simulink model "LF_V15_Delay_Perfect"  (Simulink 7.9)
settings: Solver=ode45  StartTime=0.0  StopTime=100*20e-9  RelTol=1e-3
PreLoadFcn:
  | LF_V15_Param;
values from neighbouring files (symbols this model uses):
  Cnt_CPS = 10    [LF_V15_Param.m]
  Exp_ST = 1/Exp_SF    (= 0.002)    [LF_V15_Param.m]
  Kd2 = 0.004    [LF_V15_Param.m]
  Ki2 = 0.03    [LF_V15_Param.m]
  Kp2 = 0.25    [LF_V15_Param.m]
  Reg_En = (2^Err_Acc_Len)-1    (= 511)    [LF_V15_Param.m]
  Saw_CPS = 100    [LF_V15_Param.m]
libraries: xbsIndex_r4 x273
(part 1 of 2)
settings Model: Creator=jbmervin  LastModifiedBy=Sen_Hema

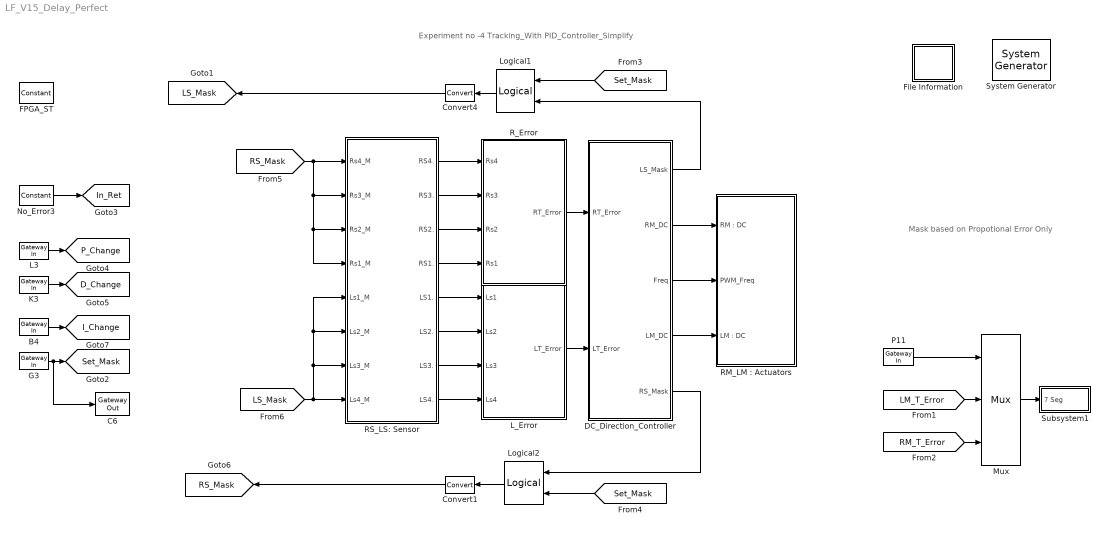
== system LF_V15_Delay_Perfect ==
  note: Experiment no -4 Tracking_With PID_Controller_Simplify
  note: Mask based on Propotional Error Only
  " System Generator" : xbsIndex_r4/ System Generator  Tag=genX  xilinxfamily=spartan3e  part=xc3s100e  speed=-4  package=cp132  synthesis_tool=XST  clock_wrapper=Clock Enables  directory=./LF_V15  proj_type=Project Navigator  Synth_file=XST Defaults  Impl_file=ISE Defaults  testbench=off  simulink_period=20e-9  sysclk_period=20  dcm_input_clock_period=10  incr_netlist=off  trim_vbits=Everywhere in SubSystem  dbl_ovrd=According to Block Masks  core_generation=According to Block Masks  run_coregen=off  deprecated_control=off  eval_field=0  block_type=sysgen
  B4 : xbsIndex_r4/Gateway In  gui_display_data_type=Boolean  arith_type=Boolean  n_bits=1  bin_pt=0  preci_type=Single  exp_width=8  frac_width=24  quantization="Round  (unbiased: +/- Inf)"  overflow=Saturate  period=InPorts_ST  dbl_ovrd=off  timing_constraint=None  locs_specified=on  LOCs={'B4'}  UseAsADC=off  ADCChannel='1'  inherit_from_input=off  hdl_port=on  block_type=gatewayin
  C6 : xbsIndex_r4/Gateway Out  inherit_from_input=off  hdl_port=on  timing_constraint=None  locs_specified=on  LOCs={'C6'}  UseAsDAC=off  DACChannel='1'  block_type=gatewayout
  Convert1 : xbsIndex_r4/Convert  gui_display_data_type=Boolean  arith_type=Boolean  n_bits=16  bin_pt=14  float_type=Single  exp_bits=8  fraction_bits=24  quantization=Truncate  overflow=Wrap  en=off  latency=0  dbl_ovrd=off  pipeline=off  block_type=convert
  Convert4 : xbsIndex_r4/Convert  gui_display_data_type=Boolean  arith_type=Boolean  n_bits=16  bin_pt=14  float_type=Single  exp_bits=8  fraction_bits=24  quantization=Truncate  overflow=Wrap  en=off  latency=0  dbl_ovrd=off  pipeline=off  block_type=convert
  DC_Direction_Controller : Subsystem
  FPGA_ST : xbsIndex_r4/Constant  const=1  gui_display_data_type=Fixed-point  arith_type=Unsigned  n_bits=1  bin_pt=0  preci_type=Single  exp_width=8  frac_width=24  explicit_period=on  period=FPGA_ST  equ=P=C  opselect=C  inp2=PCIN>>17  opr=+  inp1=P  carry=CIN  dbl_ovrd=off  block_type=constant
  File Information : Subsystem
      mask Display:
      | fprintf('','COMMENT: begin icon graphics');
      | patch([24.425 34.54 41.54 48.54 55.54 41.54 31.425 24.425 ],[32.77 32.77 39.77 32.77 39.77 39.77 39.77 32.77 ],[0.965 0.951 0.755 ]);
      | patch([31.425 41.54 34.54 24.425 31.425 ],[25.77 25.77 32.77 32.77 25.77 ],[0.95 0.93 0.15 ]);
      | patch([24.425 34.54 41.54 31.425 24.425 ],[18.77 18.77 25.77 25.77 18.77 ],[0.965 0.951 0.755 ]);
      | patch([31.425 55.54 48.54 41.54 34.54 24.425 31.425 ],[11.77 11.77 18.77 11.77 18.77 18.77 11.77 ],[0.95 0.93 0.15 ]);
      | fprintf('','COMMENT: end icon graphics');
      | fprintf('','COMMENT: end icon text');
  G3 : xbsIndex_r4/Gateway In  gui_display_data_type=Boolean  arith_type=Boolean  n_bits=1  bin_pt=0  preci_type=Single  exp_width=8  frac_width=24  quantization="Round  (unbiased: +/- Inf)"  overflow=Saturate  period=InPorts_ST  dbl_ovrd=off  timing_constraint=None  locs_specified=on  LOCs={'G3'}  UseAsADC=off  ADCChannel='1'  inherit_from_input=off  hdl_port=on  block_type=gatewayin
  K3 : xbsIndex_r4/Gateway In  gui_display_data_type=Boolean  arith_type=Boolean  n_bits=1  bin_pt=0  preci_type=Single  exp_width=8  frac_width=24  quantization="Round  (unbiased: +/- Inf)"  overflow=Saturate  period=InPorts_ST  dbl_ovrd=off  timing_constraint=None  locs_specified=on  LOCs={'K3'}  UseAsADC=off  ADCChannel='1'  inherit_from_input=off  hdl_port=on  block_type=gatewayin
  L3 : xbsIndex_r4/Gateway In  gui_display_data_type=Boolean  arith_type=Boolean  n_bits=1  bin_pt=0  preci_type=Single  exp_width=8  frac_width=24  quantization="Round  (unbiased: +/- Inf)"  overflow=Saturate  period=InPorts_ST  dbl_ovrd=off  timing_constraint=None  locs_specified=on  LOCs={'L3'}  UseAsADC=off  ADCChannel='1'  inherit_from_input=off  hdl_port=on  block_type=gatewayin
  L_Error : Subsystem
  Logical1 : xbsIndex_r4/Logical  logical_function=OR  inputs=2  en=off  latency=0  precision=User Defined  arith_type=Unsigned  n_bits=1  bin_pt=0  align_bp=on  dbl_ovrd=off  block_type=logical
  Logical2 : xbsIndex_r4/Logical  logical_function=OR  inputs=2  en=off  latency=0  precision=User Defined  arith_type=Unsigned  n_bits=1  bin_pt=0  align_bp=on  dbl_ovrd=off  block_type=logical
  Mux : xbsIndex_r4/Mux  inputs=2  en=off  latency=0  precision=Full  arith_type=Unsigned  n_bits=16  bin_pt=14  quantization=Truncate  overflow=Wrap  dbl_ovrd=off  block_type=mux
  No_Error3 : xbsIndex_r4/Constant  const=1  gui_display_data_type=Fixed-point  arith_type=Unsigned  n_bits=1  bin_pt=0  preci_type=Single  exp_width=8  frac_width=24  explicit_period=on  period=Exp_ST  equ=P=C  opselect=C  inp2=PCIN>>17  opr=+  inp1=P  carry=CIN  dbl_ovrd=off  block_type=constant
  P11 : xbsIndex_r4/Gateway In  gui_display_data_type=Boolean  arith_type=Boolean  n_bits=1  bin_pt=0  preci_type=Single  exp_width=8  frac_width=24  quantization="Round  (unbiased: +/- Inf)"  overflow=Saturate  period=20e-9  dbl_ovrd=off  timing_constraint=None  locs_specified=on  LOCs={'P11'}  UseAsADC=off  ADCChannel='1'  inherit_from_input=off  hdl_port=on  block_type=gatewayin
  "RM_LM : Actuators" : Subsystem
  RS_LS: Sensor : Subsystem
  R_Error : Subsystem
  Subsystem1 : Subsystem
  tag scope: D_Change=global, I_Change=global, In_Ret=global, LS_Mask=global, P_Change=global, RS_Mask=global, Set_Mask=global
  wires:
  RS_LS: Sensor/1(RS4.) -> R_Error/1(Rs4)
  RS_LS: Sensor/2(RS3.) -> R_Error/2(Rs3)
  RS_LS: Sensor/3(RS2.) -> R_Error/3(Rs2)
  RS_LS: Sensor/4(RS1.) -> R_Error/4(Rs1)
  RS_LS: Sensor/5(LS1.) -> L_Error/1(Ls1)
  RS_LS: Sensor/6(LS2.) -> L_Error/2(Ls2)
  RS_LS: Sensor/7(LS3.) -> L_Error/3(Ls3)
  RS_LS: Sensor/8(LS4.) -> L_Error/4(Ls4)
  DC_Direction_Controller/3(Freq) -> "RM_LM : Actuators"/2(PWM_Freq)
  DC_Direction_Controller/2(RM_DC) -> "RM_LM : Actuators"/1("RM : DC")
  DC_Direction_Controller/4(LM_DC) -> "RM_LM : Actuators"/3("LM : DC")
  R_Error/1(RT_Error) -> DC_Direction_Controller/1(RT_Error)
  L_Error/1(LT_Error) -> DC_Direction_Controller/2(LT_Error)
  DC_Direction_Controller/5(RS_Mask) -> Logical2/1
  L3/1 -> [P_Change]
  K3/1 -> [D_Change]
  B4/1 -> [I_Change]
  DC_Direction_Controller/1(LS_Mask) -> Logical1/2
  [Set_Mask] -> Logical1/1
  G3/1 -> [Set_Mask], C6/1
  [Set_Mask] -> Logical2/2
  No_Error3/1 -> [In_Ret]
  Logical1/1 -> Convert4/1
  Logical2/1 -> Convert1/1
  [RS_Mask] -> RS_LS: Sensor/1(Rs4_M), RS_LS: Sensor/2(Rs3_M), RS_LS: Sensor/3(Rs2_M), RS_LS: Sensor/4(Rs1_M)
  [LS_Mask] -> RS_LS: Sensor/8(Ls4_M), RS_LS: Sensor/7(Ls3_M), RS_LS: Sensor/5(Ls1_M), RS_LS: Sensor/6(Ls2_M)
  Convert4/1 -> [LS_Mask]
  Convert1/1 -> [RS_Mask]
  Mux/1 -> Subsystem1/1(7 Seg)
  P11/1 -> Mux/1
  [LM_T_Error] -> Mux/2
  [RM_T_Error] -> Mux/3

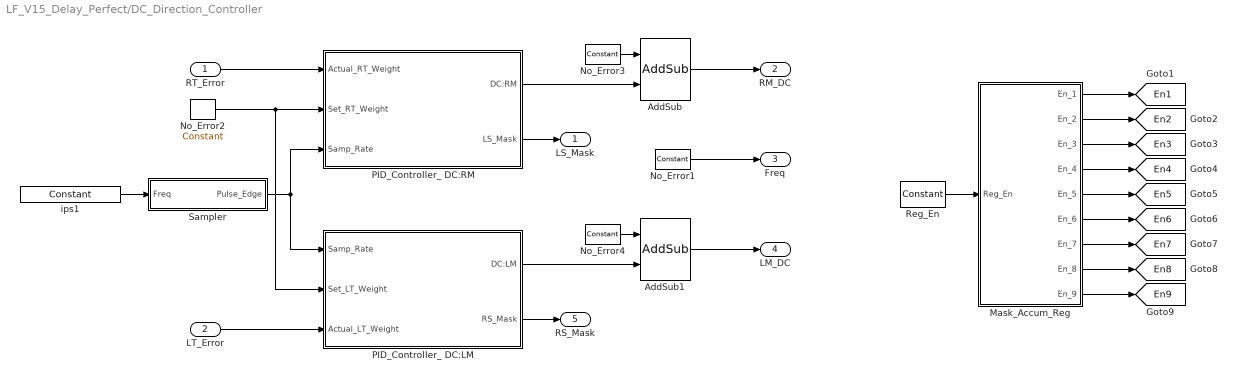
== system LF_V15_Delay_Perfect/DC_Direction_Controller ==
  RT_Error : Inport
  LT_Error : Inport  Port=2
  AddSub : xbsIndex_r4/AddSub  mode=Addition  use_carryin=off  use_carryout=off  en=off  latency=0  precision=Full  arith_type=Unsigned  n_bits=25  bin_pt=20  quantization=Truncate  overflow=Wrap  dbl_ovrd=off  use_behavioral_HDL=off  hw_selection=Fabric  pipelined=off  block_type=addsub
  AddSub1 : xbsIndex_r4/AddSub  mode=Addition  use_carryin=off  use_carryout=off  en=off  latency=0  precision=Full  arith_type=Unsigned  n_bits=25  bin_pt=20  quantization=Truncate  overflow=Wrap  dbl_ovrd=off  use_behavioral_HDL=off  hw_selection=Fabric  pipelined=off  block_type=addsub
  Mask_Accum_Reg : Subsystem
  No_Error1 : xbsIndex_r4/Constant  const=Saw_CPS  gui_display_data_type=Fixed-point  arith_type=Unsigned  n_bits=7  bin_pt=0  preci_type=Single  exp_width=8  frac_width=24  explicit_period=on  period=Exp_ST  equ=P=C  opselect=C  inp2=PCIN>>17  opr=+  inp1=P  carry=CIN  dbl_ovrd=off  block_type=constant
  No_Error2 : xbsIndex_r4/Constant  const=0  gui_display_data_type=Fixed-point  arith_type=Unsigned  n_bits=1  bin_pt=0  preci_type=Single  exp_width=8  frac_width=24  explicit_period=on  period=Exp_ST  equ=P=C  opselect=C  inp2=PCIN>>17  opr=+  inp1=P  carry=CIN  dbl_ovrd=off  block_type=constant
  No_Error3 : xbsIndex_r4/Constant  const=1  gui_display_data_type=Fixed-point  arith_type=Unsigned  n_bits=1  bin_pt=0  preci_type=Single  exp_width=8  frac_width=24  explicit_period=on  period=Exp_ST  equ=P=C  opselect=C  inp2=PCIN>>17  opr=+  inp1=P  carry=CIN  dbl_ovrd=off  block_type=constant
  No_Error4 : xbsIndex_r4/Constant  const=1  gui_display_data_type=Fixed-point  arith_type=Unsigned  n_bits=1  bin_pt=0  preci_type=Single  exp_width=8  frac_width=24  explicit_period=on  period=Exp_ST  equ=P=C  opselect=C  inp2=PCIN>>17  opr=+  inp1=P  carry=CIN  dbl_ovrd=off  block_type=constant
  PID_Controller_ DC:LM : Subsystem
  PID_Controller_ DC:RM : Subsystem
  Reg_En : xbsIndex_r4/Constant  const=Reg_En  gui_display_data_type=Fixed-point  arith_type=Unsigned  n_bits=9  bin_pt=0  preci_type=Single  exp_width=8  frac_width=24  explicit_period=on  period=Exp_ST  equ=P=C  opselect=C  inp2=PCIN>>17  opr=+  inp1=P  carry=CIN  dbl_ovrd=off  block_type=constant
  Sampler : Subsystem
  ips1 : xbsIndex_r4/Constant  const=Cnt_CPS  gui_display_data_type=Fixed-point  arith_type=Unsigned  n_bits=27  bin_pt=0  preci_type=Single  exp_width=8  frac_width=24  explicit_period=on  period=Exp_ST  equ=P=C  opselect=C  inp2=PCIN>>17  opr=+  inp1=P  carry=CIN  dbl_ovrd=off  block_type=constant
  LS_Mask : Outport
  RM_DC : Outport  Port=2
  Freq : Outport  Port=3
  LM_DC : Outport  Port=4
  RS_Mask : Outport  Port=5
  tag scope: En1=global, En2=global, En3=global, En4=global, En5=global, En6=global, En7=global, En8=global, En9=global
  wires:
  No_Error1/1 -> Freq/1
  RT_Error/1 -> PID_Controller_ DC:RM/1(Actual_RT_Weight)
  PID_Controller_ DC:RM/1(DC:RM) -> AddSub/2
  PID_Controller_ DC:LM/1(DC:LM) -> AddSub1/2
  No_Error4/1 -> AddSub1/1
  No_Error3/1 -> AddSub/1
  PID_Controller_ DC:RM/2(LS_Mask) -> LS_Mask/1
  PID_Controller_ DC:LM/2(RS_Mask) -> RS_Mask/1
  Sampler/1(Pulse_Edge) -> PID_Controller_ DC:RM/3(Samp_Rate), PID_Controller_ DC:LM/1(Samp_Rate)
  ips1/1 -> Sampler/1(Freq)
  No_Error2/1 -> PID_Controller_ DC:RM/2(Set_RT_Weight), PID_Controller_ DC:LM/2(Set_LT_Weight)
  AddSub1/1 -> LM_DC/1
  AddSub/1 -> RM_DC/1
  Mask_Accum_Reg/1(En_1) -> [En1]
  Mask_Accum_Reg/2(En_2) -> [En2]
  Mask_Accum_Reg/3(En_3) -> [En3]
  Mask_Accum_Reg/4(En_4) -> [En4]
  Mask_Accum_Reg/5(En_5) -> [En5]
  Mask_Accum_Reg/6(En_6) -> [En6]
  Mask_Accum_Reg/7(En_7) -> [En7]
  Mask_Accum_Reg/8(En_8) -> [En8]
  Mask_Accum_Reg/9(En_9) -> [En9]
  Reg_En/1 -> Mask_Accum_Reg/1("Reg_En ")
  LT_Error/1 -> PID_Controller_ DC:LM/3(Actual_LT_Weight)

== system LF_V15_Delay_Perfect/File Information ==
  note: System Identification - I ( Free Oscillation - Theta Vs Time )
  note: Expirement No -I
  note: Dynamics and Control an Enthralling Journey with Aero Thrust Pendulem
  note: _________________________________________________________________________________________________________________
  note: The Aero Thrust Pendulem is set to oscillate freely and the values of Thetas are sampled at a rate faster than the Period of oscillation
  note: Sampling Time: Sec
  note: The front end of the experiment is designed in Python by Adithya (Team Member) - This front end dynamically captures the theta and displays as a graph on the Computer Screen
      | and Simultaneously it stores the values of theta as a CSV file on the computer.  Note:  Since the initial position is considered as zero Theta. The forward positions are accounted as
      |  (1,2,3,.......60.....70....180)  and Simillarly reverse positions are accounted as (359,358......180)
  note: Method to read the CSV file
  note: Details of Front End Tool
  note: Details of Xilinx File......
  note: This Files Detrmines Theta from the Help of Signals Comming from the Encoder ( A, B, Z (not used)) and sends then theta values (datas) through all the four channels . These Channels communicate
      | the external devices through the RS232 Protocol. Simultaneously the datas are transmitted to four DAC channels Voltage ranging from ( 0V - 3.3V) for display on a CRO. In addition the datas are...
      | Displayed on a  Seven Segment LED Display avaliable on the FPGA Module...........................................................................................................................................................................................
  note: When the pendulum oscillates freely we see that the datas are recorded as ( 60....10...5....0....358.....340.....320...300) and so on .... but this will not give a visual picture of osillations
      | so we need to convert the theta as given. ( if {Theta > 180} then {Theta = (Theta - 360)}, else {Theta=Theta})...............................................................................................................

== system LF_V15_Delay_Perfect/L_Error ==
  Ls1 : Inport
  Ls2 : Inport  Port=2
  Ls3 : Inport  Port=3
  Ls4 : Inport  Port=4
  AddSub1 : xbsIndex_r4/AddSub  mode=Addition  use_carryin=off  use_carryout=off  en=off  latency=0  precision=User Defined  arith_type=Unsigned  n_bits=2  bin_pt=0  quantization=Truncate  overflow=Wrap  dbl_ovrd=off  use_behavioral_HDL=off  hw_selection=Fabric  pipelined=off  block_type=addsub
  AddSub2 : xbsIndex_r4/AddSub  mode=Addition  use_carryin=off  use_carryout=off  en=off  latency=0  precision=User Defined  arith_type=Unsigned  n_bits=4  bin_pt=0  quantization=Truncate  overflow=Wrap  dbl_ovrd=off  use_behavioral_HDL=off  hw_selection=Fabric  pipelined=off  block_type=addsub
  AddSub3 : xbsIndex_r4/AddSub  mode=Addition  use_carryin=off  use_carryout=off  en=off  latency=0  precision=User Defined  arith_type=Unsigned  n_bits=4  bin_pt=0  quantization=Truncate  overflow=Wrap  dbl_ovrd=off  use_behavioral_HDL=off  hw_selection=Fabric  pipelined=off  block_type=addsub
  LT_Error : Outport
  wires:
  AddSub2/1 -> LT_Error/1
  AddSub1/1 -> AddSub2/2
  AddSub3/1 -> AddSub2/1
  Ls1/1 -> AddSub1/2
  Ls2/1 -> AddSub1/1
  Ls3/1 -> AddSub3/2
  Ls4/1 -> AddSub3/1

== system LF_V15_Delay_Perfect/RM_LM : Actuators ==
  "RM : DC" : Inport
  PWM_Freq : Inport  Port=2
  "LM : DC" : Inport  Port=3
  L_Actuator : Subsystem
  RM_LM: F_R_PWM_Generator : Subsystem
  R_Actuators : Subsystem
  wires:
  "RM : DC"/1 -> RM_LM: F_R_PWM_Generator/1(RM:DC)
  "LM : DC"/1 -> RM_LM: F_R_PWM_Generator/2(LM:DC)
  PWM_Freq/1 -> RM_LM: F_R_PWM_Generator/3(RM_LM:PWM_Freq)
  RM_LM: F_R_PWM_Generator/1(RM: F_PWM) -> R_Actuators/1("RM : F_PWM")
  RM_LM: F_R_PWM_Generator/4(LM: F_PWM) -> L_Actuator/2(LM: F_PWM)
  RM_LM: F_R_PWM_Generator/3(LM: R_PWM) -> L_Actuator/1(LM: R_PWM)
  RM_LM: F_R_PWM_Generator/2(RM: R_PWM) -> R_Actuators/2(RM :R_ PWM)

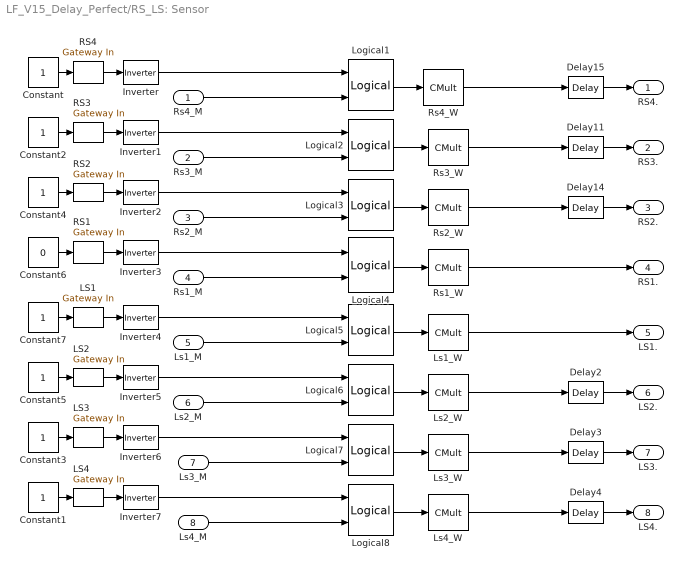
== system LF_V15_Delay_Perfect/RS_LS: Sensor ==
  Rs4_M : Inport
  Rs3_M : Inport  Port=2
  Rs2_M : Inport  Port=3
  Rs1_M : Inport  Port=4
  Ls1_M : Inport  Port=5
  Ls2_M : Inport  Port=6
  Ls3_M : Inport  Port=7
  Ls4_M : Inport  Port=8
  Constant{,1..5,7} (7 alike) : Constant
  Constant6 : Constant  Value=0
  Delay11 : xbsIndex_r4/Delay  rst=off  infoeditControl=Selection of Reset will increase slice count due to use of real FFs and instead of SRLs  en=off  latency=RSLS3_D  dbl_ovrd=off  reg_retiming=off  block_type=delay
  Delay14 : xbsIndex_r4/Delay  rst=off  infoeditControl=Selection of Reset will increase slice count due to use of real FFs and instead of SRLs  en=off  latency=RSLS2_D  dbl_ovrd=off  reg_retiming=off  block_type=delay
  Delay15 : xbsIndex_r4/Delay  rst=off  infoeditControl=Selection of Reset will increase slice count due to use of real FFs and instead of SRLs  en=off  latency=RSLS4_D  dbl_ovrd=off  reg_retiming=off  block_type=delay
  Delay2 : xbsIndex_r4/Delay  rst=off  infoeditControl=Selection of Reset will increase slice count due to use of real FFs and instead of SRLs  en=off  latency=RSLS2_D  dbl_ovrd=off  reg_retiming=off  block_type=delay
  Delay3 : xbsIndex_r4/Delay  rst=off  infoeditControl=Selection of Reset will increase slice count due to use of real FFs and instead of SRLs  en=off  latency=RSLS3_D  dbl_ovrd=off  reg_retiming=off  block_type=delay
  Delay4 : xbsIndex_r4/Delay  rst=off  infoeditControl=Selection of Reset will increase slice count due to use of real FFs and instead of SRLs  en=off  latency=RSLS4_D  dbl_ovrd=off  reg_retiming=off  block_type=delay
  Inverter{,1..7} (8 alike) : xbsIndex_r4/Inverter  en=off  latency=0  dbl_ovrd=off  block_type=inv
  LS1 : xbsIndex_r4/Gateway In  gui_display_data_type=Boolean  arith_type=Boolean  n_bits=1  bin_pt=0  preci_type=Single  exp_width=8  frac_width=24  quantization="Round  (unbiased: +/- Inf)"  overflow=Saturate  period=InPorts_ST  dbl_ovrd=off  timing_constraint=None  locs_specified=on  LOCs={'A9'}  UseAsADC=off  ADCChannel='1'  inherit_from_input=off  hdl_port=on  block_type=gatewayin
  LS2 : xbsIndex_r4/Gateway In  gui_display_data_type=Boolean  arith_type=Boolean  n_bits=1  bin_pt=0  preci_type=Single  exp_width=8  frac_width=24  quantization="Round  (unbiased: +/- Inf)"  overflow=Saturate  period=InPorts_ST  dbl_ovrd=off  timing_constraint=None  locs_specified=on  LOCs={'B7'}  UseAsADC=off  ADCChannel='1'  inherit_from_input=off  hdl_port=on  block_type=gatewayin
  LS3 : xbsIndex_r4/Gateway In  gui_display_data_type=Boolean  arith_type=Boolean  n_bits=1  bin_pt=0  preci_type=Single  exp_width=8  frac_width=24  quantization="Round  (unbiased: +/- Inf)"  overflow=Saturate  period=InPorts_ST  dbl_ovrd=off  timing_constraint=None  locs_specified=on  LOCs={'C5'}  UseAsADC=off  ADCChannel='1'  inherit_from_input=off  hdl_port=on  block_type=gatewayin
  LS4 : xbsIndex_r4/Gateway In  gui_display_data_type=Boolean  arith_type=Boolean  n_bits=1  bin_pt=0  preci_type=Single  exp_width=8  frac_width=24  quantization="Round  (unbiased: +/- Inf)"  overflow=Saturate  period=InPorts_ST  dbl_ovrd=off  timing_constraint=None  locs_specified=on  LOCs={'B6'}  UseAsADC=off  ADCChannel='1'  inherit_from_input=off  hdl_port=on  block_type=gatewayin
  Logical{1..8} (8 alike) : xbsIndex_r4/Logical  logical_function=AND  inputs=2  en=off  latency=0  precision=User Defined  arith_type=Unsigned  n_bits=1  bin_pt=0  align_bp=on  dbl_ovrd=off  block_type=logical
  Ls1_W : xbsIndex_r4/CMult  const=1  gui_display_data_type=Fixed-point  const_n_bits=1  const_bin_pt=0  float_type=Single  exp_bits=8  fraction_bits=24  en=off  latency=0  precision=User Defined  arith_type=Unsigned  n_bits=1  bin_pt=0  quantization=Truncate  overflow=Wrap  dbl_ovrd=off  use_behavioral_HDL=off  mem_type=Distributed RAM  pipeline=off  block_type=cmult
  Ls2_W : xbsIndex_r4/CMult  const=2  gui_display_data_type=Fixed-point  const_n_bits=2  const_bin_pt=0  float_type=Single  exp_bits=8  fraction_bits=24  en=off  latency=0  precision=User Defined  arith_type=Unsigned  n_bits=2  bin_pt=0  quantization=Truncate  overflow=Wrap  dbl_ovrd=off  use_behavioral_HDL=off  mem_type=Distributed RAM  pipeline=off  block_type=cmult
  Ls3_W : xbsIndex_r4/CMult  const=4  gui_display_data_type=Fixed-point  const_n_bits=3  const_bin_pt=0  float_type=Single  exp_bits=8  fraction_bits=24  en=off  latency=0  precision=User Defined  arith_type=Unsigned  n_bits=3  bin_pt=0  quantization=Truncate  overflow=Wrap  dbl_ovrd=off  use_behavioral_HDL=off  mem_type=Distributed RAM  pipeline=off  block_type=cmult
  Ls4_W : xbsIndex_r4/CMult  const=8  gui_display_data_type=Fixed-point  const_n_bits=4  const_bin_pt=0  float_type=Single  exp_bits=8  fraction_bits=24  en=off  latency=0  precision=User Defined  arith_type=Unsigned  n_bits=4  bin_pt=0  quantization=Truncate  overflow=Wrap  dbl_ovrd=off  use_behavioral_HDL=off  mem_type=Distributed RAM  pipeline=off  block_type=cmult
  RS1 : xbsIndex_r4/Gateway In  gui_display_data_type=Boolean  arith_type=Boolean  n_bits=1  bin_pt=0  preci_type=Single  exp_width=8  frac_width=24  quantization="Round  (unbiased: +/- Inf)"  overflow=Saturate  period=InPorts_ST  dbl_ovrd=off  timing_constraint=None  locs_specified=on  LOCs={'B9'}  UseAsADC=off  ADCChannel='1'  inherit_from_input=off  hdl_port=on  block_type=gatewayin
  RS2 : xbsIndex_r4/Gateway In  gui_display_data_type=Boolean  arith_type=Boolean  n_bits=1  bin_pt=0  preci_type=Single  exp_width=8  frac_width=24  quantization="Round  (unbiased: +/- Inf)"  overflow=Saturate  period=InPorts_ST  dbl_ovrd=off  timing_constraint=None  locs_specified=on  LOCs={'A10'}  UseAsADC=off  ADCChannel='1'  inherit_from_input=off  hdl_port=on  block_type=gatewayin
  RS3 : xbsIndex_r4/Gateway In  gui_display_data_type=Boolean  arith_type=Boolean  n_bits=1  bin_pt=0  preci_type=Single  exp_width=8  frac_width=24  quantization="Round  (unbiased: +/- Inf)"  overflow=Saturate  period=InPorts_ST  dbl_ovrd=off  timing_constraint=None  locs_specified=on  LOCs={'C9'}  UseAsADC=off  ADCChannel='1'  inherit_from_input=off  hdl_port=on  block_type=gatewayin
  RS4 : xbsIndex_r4/Gateway In  gui_display_data_type=Boolean  arith_type=Boolean  n_bits=1  bin_pt=0  preci_type=Single  exp_width=8  frac_width=24  quantization="Round  (unbiased: +/- Inf)"  overflow=Saturate  period=InPorts_ST  dbl_ovrd=off  timing_constraint=None  locs_specified=on  LOCs={'C12'}  UseAsADC=off  ADCChannel='1'  inherit_from_input=off  hdl_port=on  block_type=gatewayin
  Rs1_W : xbsIndex_r4/CMult  const=1  gui_display_data_type=Fixed-point  const_n_bits=1  const_bin_pt=0  float_type=Single  exp_bits=8  fraction_bits=24  en=off  latency=0  precision=User Defined  arith_type=Unsigned  n_bits=1  bin_pt=0  quantization=Truncate  overflow=Wrap  dbl_ovrd=off  use_behavioral_HDL=off  mem_type=Distributed RAM  pipeline=off  block_type=cmult
  Rs2_W : xbsIndex_r4/CMult  const=2  gui_display_data_type=Fixed-point  const_n_bits=2  const_bin_pt=0  float_type=Single  exp_bits=8  fraction_bits=24  en=off  latency=0  precision=User Defined  arith_type=Unsigned  n_bits=2  bin_pt=0  quantization=Truncate  overflow=Wrap  dbl_ovrd=off  use_behavioral_HDL=off  mem_type=Distributed RAM  pipeline=off  block_type=cmult
  Rs3_W : xbsIndex_r4/CMult  const=4  gui_display_data_type=Fixed-point  const_n_bits=3  const_bin_pt=0  float_type=Single  exp_bits=8  fraction_bits=24  en=off  latency=0  precision=User Defined  arith_type=Unsigned  n_bits=3  bin_pt=0  quantization=Truncate  overflow=Wrap  dbl_ovrd=off  use_behavioral_HDL=off  mem_type=Distributed RAM  pipeline=off  block_type=cmult
  Rs4_W : xbsIndex_r4/CMult  const=8  gui_display_data_type=Fixed-point  const_n_bits=4  const_bin_pt=0  float_type=Single  exp_bits=8  fraction_bits=24  en=off  latency=0  precision=User Defined  arith_type=Unsigned  n_bits=4  bin_pt=0  quantization=Truncate  overflow=Wrap  dbl_ovrd=off  use_behavioral_HDL=off  mem_type=Distributed RAM  pipeline=off  block_type=cmult
  RS4. : Outport
  RS3. : Outport  Port=2
  RS2. : Outport  Port=3
  RS1. : Outport  Port=4
  LS1. : Outport  Port=5
  LS2. : Outport  Port=6
  LS3. : Outport  Port=7
  LS4. : Outport  Port=8
  wires:
  RS4/1 -> Inverter/1
  RS3/1 -> Inverter1/1
  RS2/1 -> Inverter2/1
  RS1/1 -> Inverter3/1
  LS1/1 -> Inverter4/1
  LS2/1 -> Inverter5/1
  LS3/1 -> Inverter6/1
  LS4/1 -> Inverter7/1
  Inverter/1 -> Logical1/1
  Logical1/1 -> Rs4_W/1
  Rs4_M/1 -> Logical1/2
  Rs3_M/1 -> Logical2/2
  Logical2/1 -> Rs3_W/1
  Inverter1/1 -> Logical2/1
  Rs2_M/1 -> Logical3/2
  Inverter2/1 -> Logical3/1
  Logical3/1 -> Rs2_W/1
  Rs1_M/1 -> Logical4/2
  Inverter3/1 -> Logical4/1
  Logical4/1 -> Rs1_W/1
  Ls1_M/1 -> Logical5/2
  Inverter4/1 -> Logical5/1
  Ls2_M/1 -> Logical6/2
  Inverter5/1 -> Logical6/1
  Ls3_M/1 -> Logical7/2
  Inverter6/1 -> Logical7/1
  Ls4_M/1 -> Logical8/2
  Inverter7/1 -> Logical8/1
  Logical5/1 -> Ls1_W/1
  Logical6/1 -> Ls2_W/1
  Logical7/1 -> Ls3_W/1
  Logical8/1 -> Ls4_W/1
  Constant/1 -> RS4/1
  Constant1/1 -> LS4/1
  Constant2/1 -> RS3/1
  Constant3/1 -> LS3/1
  Constant4/1 -> RS2/1
  Constant5/1 -> LS2/1
  Constant6/1 -> RS1/1
  Constant7/1 -> LS1/1
  Rs3_W/1 -> Delay11/1
  Ls4_W/1 -> Delay4/1
  Ls3_W/1 -> Delay3/1
  Rs2_W/1 -> Delay14/1
  Ls2_W/1 -> Delay2/1
  Rs1_W/1 -> RS1./1
  Ls1_W/1 -> LS1./1
  Rs4_W/1 -> Delay15/1
  Delay11/1 -> RS3./1
  Delay3/1 -> LS3./1
  Delay2/1 -> LS2./1
  Delay14/1 -> RS2./1
  Delay15/1 -> RS4./1
  Delay4/1 -> LS4./1

== system LF_V15_Delay_Perfect/R_Error ==
  Rs4 : Inport
  Rs3 : Inport  Port=2
  Rs2 : Inport  Port=3
  Rs1 : Inport  Port=4
  AddSub1 : xbsIndex_r4/AddSub  mode=Addition  use_carryin=off  use_carryout=off  en=off  latency=0  precision=User Defined  arith_type=Unsigned  n_bits=2  bin_pt=0  quantization=Truncate  overflow=Wrap  dbl_ovrd=off  use_behavioral_HDL=off  hw_selection=Fabric  pipelined=off  block_type=addsub
  AddSub2 : xbsIndex_r4/AddSub  mode=Addition  use_carryin=off  use_carryout=off  en=off  latency=0  precision=User Defined  arith_type=Unsigned  n_bits=4  bin_pt=0  quantization=Truncate  overflow=Wrap  dbl_ovrd=off  use_behavioral_HDL=off  hw_selection=Fabric  pipelined=off  block_type=addsub
  AddSub3 : xbsIndex_r4/AddSub  mode=Addition  use_carryin=off  use_carryout=off  en=off  latency=0  precision=User Defined  arith_type=Unsigned  n_bits=4  bin_pt=0  quantization=Truncate  overflow=Wrap  dbl_ovrd=off  use_behavioral_HDL=off  hw_selection=Fabric  pipelined=off  block_type=addsub
  RT_Error : Outport
  wires:
  Rs4/1 -> AddSub3/1
  Rs3/1 -> AddSub3/2
  AddSub2/1 -> RT_Error/1
  Rs2/1 -> AddSub1/1
  Rs1/1 -> AddSub1/2
  AddSub1/1 -> AddSub2/2
  AddSub3/1 -> AddSub2/1

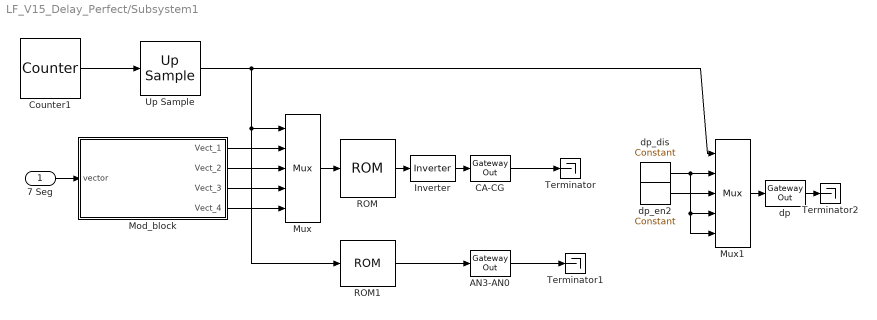
== system LF_V15_Delay_Perfect/Subsystem1 ==
  7 Seg : Inport
  AN3-AN0 : xbsIndex_r4/Gateway Out  inherit_from_input=off  hdl_port=on  timing_constraint=None  locs_specified=on  LOCs={'K14','M13','J12','F12'}  UseAsDAC=off  DACChannel='1'  block_type=gatewayout
  CA-CG : xbsIndex_r4/Gateway Out  inherit_from_input=off  hdl_port=on  timing_constraint=None  locs_specified=on  LOCs={'L14','H12','N14','N11','P12','L13','M12'}  UseAsDAC=off  DACChannel='1'  block_type=gatewayout
  Counter1 : xbsIndex_r4/Counter  cnt_type=Count Limited  cnt_to=3  operation=Up  start_count=0  cnt_by_val=1  arith_type=Unsigned  n_bits=2  bin_pt=0  load_pin=off  rst=off  en=off  explicit_period=on  period=20e-5  dbl_ovrd=off  use_behavioral_HDL=off  implementation=Fabric  block_type=counter
  Inverter : xbsIndex_r4/Inverter  en=off  latency=0  dbl_ovrd=off  block_type=inv
  Mod_block : Subsystem
  Mux : xbsIndex_r4/Mux  inputs=4  en=off  latency=0  precision=User Defined  arith_type=Unsigned  n_bits=4  bin_pt=0  quantization=Truncate  overflow=Wrap  dbl_ovrd=off  block_type=mux
  Mux1 : xbsIndex_r4/Mux  inputs=4  en=off  latency=0  precision=User Defined  arith_type=Unsigned  n_bits=1  bin_pt=0  quantization=Truncate  overflow=Wrap  dbl_ovrd=off  block_type=mux
  ROM : xbsIndex_r4/ROM  depth=10  initVector="[126 48 109 121 51 91 95 112 127  123]"  distributed_mem=Distributed memory  rst=off  init_reg=0  en=off  latency=0  gui_display_data_type=Fixed-point  arith_type=Unsigned  n_bits=7  bin_pt=0  preci_type=Single  exp_width=8  frac_width=24  dbl_ovrd=off  optimize=Area  use_rpm=on  block_type=sprom
  ROM1 : xbsIndex_r4/ROM  depth=4  initVector=[7 11 13 14]  distributed_mem=Distributed memory  rst=off  init_reg=0  en=off  latency=0  gui_display_data_type=Fixed-point  arith_type=Unsigned  n_bits=4  bin_pt=0  preci_type=Single  exp_width=8  frac_width=24  dbl_ovrd=off  optimize=Area  use_rpm=on  block_type=sprom
  Terminator : Terminator
  Terminator1 : Terminator
  Terminator2 : Terminator
  Up Sample : xbsIndex_r4/Up Sample  sample_ratio=10000  copy_samples=on  en=off  latency=0  dbl_ovrd=off  block_type=usamp
  dp : xbsIndex_r4/Gateway Out  inherit_from_input=off  hdl_port=on  timing_constraint=None  locs_specified=on  LOCs={'N13'}  UseAsDAC=off  DACChannel='1'  block_type=gatewayout
  dp_dis : xbsIndex_r4/Constant  const=1  gui_display_data_type=Fixed-point  arith_type=Unsigned  n_bits=1  bin_pt=0  preci_type=Single  exp_width=8  frac_width=24  explicit_period=on  period=20e-9  equ=P=C  opselect=C  inp2=PCIN>>17  opr=+  inp1=P  carry=CIN  dbl_ovrd=off  block_type=constant
  dp_en2 : xbsIndex_r4/Constant  const=0  gui_display_data_type=Fixed-point  arith_type=Unsigned  n_bits=1  bin_pt=0  preci_type=Single  exp_width=8  frac_width=24  explicit_period=on  period=20e-9  equ=P=C  opselect=C  inp2=PCIN>>17  opr=+  inp1=P  carry=CIN  dbl_ovrd=off  block_type=constant
  wires:
  dp/1 -> Terminator2/1
  CA-CG/1 -> Terminator/1
  AN3-AN0/1 -> Terminator1/1
  Up Sample/1 -> Mux/1, ROM1/1, Mux1/1
  ROM1/1 -> AN3-AN0/1
  Mux/1 -> ROM/1
  Mod_block/4(Vect_4) -> Mux/5
  Mod_block/3(Vect_3) -> Mux/4
  Mod_block/2(Vect_2) -> Mux/3
  Mod_block/1(Vect_1) -> Mux/2
  Inverter/1 -> CA-CG/1
  ROM/1 -> Inverter/1
  Counter1/1 -> Up Sample/1
  7 Seg/1 -> Mod_block/1(vector)
  Mux1/1 -> dp/1
  dp_dis/1 -> Mux1/2, Mux1/4, Mux1/5
  dp_en2/1 -> Mux1/3

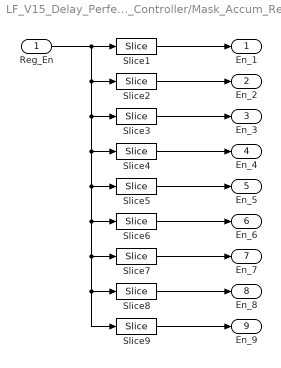
== system LF_V15_Delay_Perfect/DC_Direction_Controller/Mask_Accum_Reg ==
  "Reg_En " : Inport
  Slice1 : xbsIndex_r4/Slice  nbits=1  boolean_output=on  mode=Lower Bit Location + Width  bit1=0  base1=MSB of Input  bit0=0  base0=LSB of Input  dbl_ovrd=off  block_type=slice
  Slice2 : xbsIndex_r4/Slice  nbits=1  boolean_output=on  mode=Lower Bit Location + Width  bit1=0  base1=MSB of Input  bit0=1  base0=LSB of Input  dbl_ovrd=off  block_type=slice
  Slice3 : xbsIndex_r4/Slice  nbits=1  boolean_output=on  mode=Lower Bit Location + Width  bit1=0  base1=MSB of Input  bit0=2  base0=LSB of Input  dbl_ovrd=off  block_type=slice
  Slice4 : xbsIndex_r4/Slice  nbits=1  boolean_output=on  mode=Lower Bit Location + Width  bit1=0  base1=MSB of Input  bit0=3  base0=LSB of Input  dbl_ovrd=off  block_type=slice
  Slice5 : xbsIndex_r4/Slice  nbits=1  boolean_output=on  mode=Lower Bit Location + Width  bit1=0  base1=MSB of Input  bit0=4  base0=LSB of Input  dbl_ovrd=off  block_type=slice
  Slice6 : xbsIndex_r4/Slice  nbits=1  boolean_output=on  mode=Lower Bit Location + Width  bit1=0  base1=MSB of Input  bit0=5  base0=LSB of Input  dbl_ovrd=off  block_type=slice
  Slice7 : xbsIndex_r4/Slice  nbits=1  boolean_output=on  mode=Lower Bit Location + Width  bit1=0  base1=MSB of Input  bit0=6  base0=LSB of Input  dbl_ovrd=off  block_type=slice
  Slice8 : xbsIndex_r4/Slice  nbits=1  boolean_output=on  mode=Lower Bit Location + Width  bit1=0  base1=MSB of Input  bit0=7  base0=LSB of Input  dbl_ovrd=off  block_type=slice
  Slice9 : xbsIndex_r4/Slice  nbits=1  boolean_output=on  mode=Lower Bit Location + Width  bit1=0  base1=MSB of Input  bit0=8  base0=LSB of Input  dbl_ovrd=off  block_type=slice
  En_1 : Outport
  En_2 : Outport  Port=2
  En_3 : Outport  Port=3
  En_4 : Outport  Port=4
  En_5 : Outport  Port=5
  En_6 : Outport  Port=6
  En_7 : Outport  Port=7
  En_8 : Outport  Port=8
  En_9 : Outport  Port=9
  wires:
  "Reg_En "/1 -> Slice5/1, Slice6/1, Slice9/1, Slice8/1, Slice7/1, Slice4/1, Slice3/1, Slice2/1, Slice1/1
  Slice1/1 -> En_1/1
  Slice2/1 -> En_2/1
  Slice3/1 -> En_3/1
  Slice4/1 -> En_4/1
  Slice5/1 -> En_5/1
  Slice6/1 -> En_6/1
  Slice7/1 -> En_7/1
  Slice8/1 -> En_8/1
  Slice9/1 -> En_9/1

== system LF_V15_Delay_Perfect/DC_Direction_Controller/PID_Controller_ DC:LM ==
  Samp_Rate : Inport
  Set_LT_Weight : Inport  Port=2
  Actual_LT_Weight : Inport  Port=3
  AddSub : xbsIndex_r4/AddSub  mode=Subtraction  use_carryin=off  use_carryout=off  en=off  latency=0  precision=User Defined  arith_type="Signed  (2's comp)"  n_bits=5  bin_pt=0  quantization=Truncate  overflow=Wrap  dbl_ovrd=off  use_behavioral_HDL=off  hw_selection=Fabric  pipelined=off  block_type=addsub
  AddSub2 : xbsIndex_r4/AddSub  mode=Addition  use_carryin=off  use_carryout=off  en=off  latency=0  precision=Full  arith_type="Signed  (2's comp)"  n_bits=25  bin_pt=20  quantization=Truncate  overflow=Wrap  dbl_ovrd=off  use_behavioral_HDL=off  hw_selection=Fabric  pipelined=off  block_type=addsub
  ID_Controller : Subsystem
  P_Controller : Subsystem
  RS_Mask_Control : Subsystem
  DC:LM : Outport
  RS_Mask : Outport  Port=2
  wires:
  Samp_Rate/1 -> ID_Controller/2(Samp_Rate)
  RS_Mask_Control/1(RS_Mask) -> RS_Mask/1
  AddSub2/1 -> DC:LM/1
  P_Controller/1(P_Out) -> AddSub2/1
  ID_Controller/1(ID_Out) -> AddSub2/2
  Actual_LT_Weight/1 -> AddSub/2
  Set_LT_Weight/1 -> AddSub/1
  AddSub/1 -> ID_Controller/1(Error), P_Controller/1(Err)

== system LF_V15_Delay_Perfect/DC_Direction_Controller/PID_Controller_ DC:RM ==
  Actual_RT_Weight : Inport
  Set_RT_Weight : Inport  Port=2
  Samp_Rate : Inport  Port=3
  AddSub : xbsIndex_r4/AddSub  mode=Subtraction  use_carryin=off  use_carryout=off  en=off  latency=0  precision=User Defined  arith_type="Signed  (2's comp)"  n_bits=5  bin_pt=0  quantization=Truncate  overflow=Wrap  dbl_ovrd=off  use_behavioral_HDL=off  hw_selection=Fabric  pipelined=off  block_type=addsub
  AddSub2 : xbsIndex_r4/AddSub  mode=Addition  use_carryin=off  use_carryout=off  en=off  latency=0  precision=Full  arith_type="Signed  (2's comp)"  n_bits=25  bin_pt=20  quantization=Truncate  overflow=Wrap  dbl_ovrd=off  use_behavioral_HDL=off  hw_selection=Fabric  pipelined=off  block_type=addsub
  ID_Controller : Subsystem
  LS_Mask_Control : Subsystem
  P_Controller : Subsystem
  DC:RM : Outport
  LS_Mask : Outport  Port=2
  wires:
  AddSub/1 -> P_Controller/1(Err), ID_Controller/1(Error)
  Set_RT_Weight/1 -> AddSub/1
  Actual_RT_Weight/1 -> AddSub/2
  ID_Controller/1(ID_Out) -> AddSub2/2
  P_Controller/1(P_Out) -> AddSub2/1
  LS_Mask_Control/1(LS_Mask) -> LS_Mask/1
  Samp_Rate/1 -> ID_Controller/2(Samp_Rate)
  AddSub2/1 -> DC:RM/1

== system LF_V15_Delay_Perfect/DC_Direction_Controller/Sampler ==
  Freq : Inport
  Convert2 : xbsIndex_r4/Convert  gui_display_data_type=Boolean  arith_type=Boolean  n_bits=16  bin_pt=14  float_type=Single  exp_bits=8  fraction_bits=24  quantization=Truncate  overflow=Wrap  en=off  latency=0  dbl_ovrd=off  pipeline=off  block_type=convert
  Convert4 : xbsIndex_r4/Convert  gui_display_data_type=Boolean  arith_type=Boolean  n_bits=16  bin_pt=14  float_type=Single  exp_bits=8  fraction_bits=24  quantization=Truncate  overflow=Wrap  en=off  latency=0  dbl_ovrd=off  pipeline=off  block_type=convert
  Pulse_generator : Subsystem
  Subsystem1 : Subsystem
      mask Display: disp('Edge\nDetection');
  Pulse_Edge : Outport
  wires:
  Freq/1 -> Pulse_generator/1(Freq)
  Convert2/1 -> Pulse_Edge/1
  Pulse_generator/1(Pulse_Level) -> Convert4/1
  Convert4/1 -> Subsystem1/1(In1)
  Subsystem1/1(Out1) -> Convert2/1

== system LF_V15_Delay_Perfect/RM_LM : Actuators/L_Actuator ==
  LM: R_PWM : Inport
  LM: F_PWM : Inport  Port=2
  LM_N : xbsIndex_r4/Gateway Out  inherit_from_input=off  hdl_port=on  timing_constraint=None  locs_specified=on  LOCs={'J3'}  UseAsDAC=off  DACChannel='1'  block_type=gatewayout
  LM_P : xbsIndex_r4/Gateway Out  inherit_from_input=off  hdl_port=on  timing_constraint=None  locs_specified=on  LOCs={'B5'}  UseAsDAC=off  DACChannel='1'  block_type=gatewayout
  wires:
  LM: F_PWM/1 -> LM_P/1
  LM: R_PWM/1 -> LM_N/1

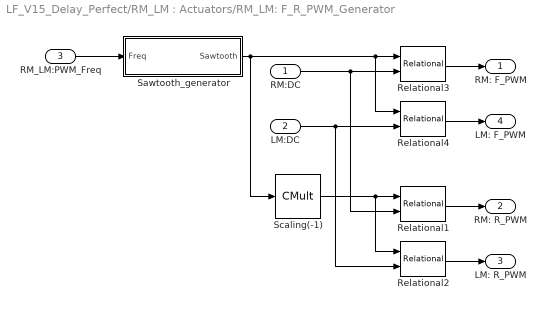
== system LF_V15_Delay_Perfect/RM_LM : Actuators/RM_LM: F_R_PWM_Generator ==
  RM:DC : Inport
  LM:DC : Inport  Port=2
  RM_LM:PWM_Freq : Inport  Port=3
  Relational1 : xbsIndex_r4/Relational  mode=a>b  en=off  latency=0  dbl_ovrd=off  block_type=relational
  Relational2 : xbsIndex_r4/Relational  mode=a>b  en=off  latency=0  dbl_ovrd=off  block_type=relational
  Relational3 : xbsIndex_r4/Relational  mode=a<b  en=off  latency=0  dbl_ovrd=off  block_type=relational
  Relational4 : xbsIndex_r4/Relational  mode=a<b  en=off  latency=0  dbl_ovrd=off  block_type=relational
  Sawtooth_generator : Subsystem
  Scaling(-1) : xbsIndex_r4/CMult  const=-1  gui_display_data_type=Fixed-point  const_n_bits=2  const_bin_pt=0  float_type=Single  exp_bits=8  fraction_bits=24  en=off  latency=0  precision=Full  arith_type=Unsigned  n_bits=21  bin_pt=20  quantization=Truncate  overflow=Wrap  dbl_ovrd=off  use_behavioral_HDL=on  mem_type=Distributed RAM  pipeline=off  block_type=cmult
  RM: F_PWM : Outport
  RM: R_PWM : Outport  Port=2
  LM: R_PWM : Outport  Port=3
  LM: F_PWM : Outport  Port=4
  wires:
  Relational3/1 -> RM: F_PWM/1
  RM_LM:PWM_Freq/1 -> Sawtooth_generator/1(Freq)
  Relational4/1 -> LM: F_PWM/1
  Sawtooth_generator/1(Sawtooth) -> Relational3/1, Relational4/1, Scaling(-1)/1
  RM:DC/1 -> Relational3/2, Relational1/2
  LM:DC/1 -> Relational2/2, Relational4/2
  Scaling(-1)/1 -> Relational2/1, Relational1/1
  Relational1/1 -> RM: R_PWM/1
  Relational2/1 -> LM: R_PWM/1

== system LF_V15_Delay_Perfect/RM_LM : Actuators/R_Actuators ==
  "RM : F_PWM" : Inport
  RM :R_ PWM : Inport  Port=2
  RM_N : xbsIndex_r4/Gateway Out  inherit_from_input=off  hdl_port=on  timing_constraint=None  locs_specified=on  LOCs={'B2'}  UseAsDAC=off  DACChannel='1'  block_type=gatewayout
  RM_P : xbsIndex_r4/Gateway Out  inherit_from_input=off  hdl_port=on  timing_constraint=None  locs_specified=on  LOCs={'A3'}  UseAsDAC=off  DACChannel='1'  block_type=gatewayout
  wires:
  "RM : F_PWM"/1 -> RM_P/1
  RM :R_ PWM/1 -> RM_N/1

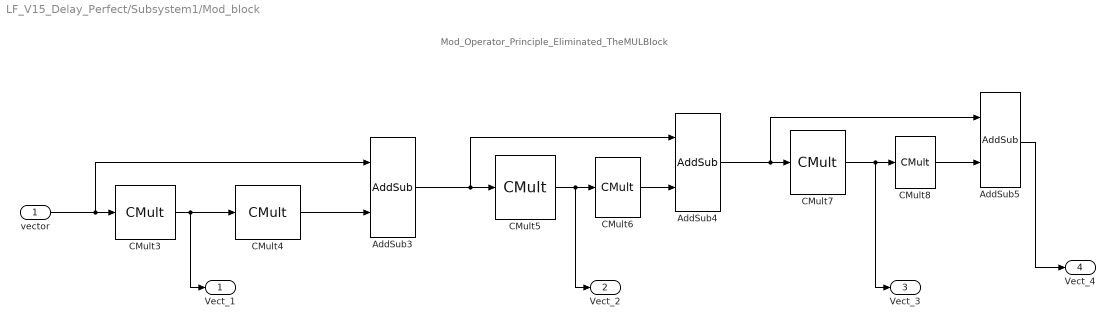
== system LF_V15_Delay_Perfect/Subsystem1/Mod_block ==
  note: Mod_Operator_Principle_Eliminated_TheMULBlock
  vector : Inport
  AddSub3 : xbsIndex_r4/AddSub  mode=Subtraction  use_carryin=off  use_carryout=off  en=off  latency=0  precision=User Defined  arith_type=Unsigned  n_bits=10  bin_pt=0  quantization=Truncate  overflow=Wrap  dbl_ovrd=off  use_behavioral_HDL=off  hw_selection=Fabric  pipelined=off  block_type=addsub
  AddSub4 : xbsIndex_r4/AddSub  mode=Subtraction  use_carryin=off  use_carryout=off  en=off  latency=0  precision=User Defined  arith_type=Unsigned  n_bits=7  bin_pt=0  quantization=Truncate  overflow=Saturate  dbl_ovrd=off  use_behavioral_HDL=off  hw_selection=Fabric  pipelined=off  block_type=addsub
  AddSub5 : xbsIndex_r4/AddSub  mode=Subtraction  use_carryin=off  use_carryout=off  en=off  latency=0  precision=User Defined  arith_type=Unsigned  n_bits=4  bin_pt=0  quantization=Truncate  overflow=Saturate  dbl_ovrd=off  use_behavioral_HDL=off  hw_selection=Fabric  pipelined=off  block_type=addsub
  CMult3 : xbsIndex_r4/CMult  const=0.001  gui_display_data_type=Fixed-point  const_n_bits=30  const_bin_pt=30  float_type=Single  exp_bits=8  fraction_bits=24  en=off  latency=0  precision=User Defined  arith_type=Unsigned  n_bits=4  bin_pt=0  quantization=Truncate  overflow=Wrap  dbl_ovrd=off  use_behavioral_HDL=off  mem_type=Distributed RAM  pipeline=off  block_type=cmult
  CMult4 : xbsIndex_r4/CMult  const=1000  gui_display_data_type=Fixed-point  const_n_bits=10  const_bin_pt=0  float_type=Single  exp_bits=8  fraction_bits=24  en=off  latency=0  precision=User Defined  arith_type=Unsigned  n_bits=15  bin_pt=0  quantization=Truncate  overflow=Wrap  dbl_ovrd=off  use_behavioral_HDL=off  mem_type=Distributed RAM  pipeline=off  block_type=cmult
  CMult5 : xbsIndex_r4/CMult  const=0.01  gui_display_data_type=Fixed-point  const_n_bits=20  const_bin_pt=20  float_type=Single  exp_bits=8  fraction_bits=24  en=off  latency=0  precision=User Defined  arith_type=Unsigned  n_bits=4  bin_pt=0  quantization=Truncate  overflow=Saturate  dbl_ovrd=off  use_behavioral_HDL=off  mem_type=Distributed RAM  pipeline=off  block_type=cmult
  CMult6 : xbsIndex_r4/CMult  const=100  gui_display_data_type=Fixed-point  const_n_bits=7  const_bin_pt=0  float_type=Single  exp_bits=8  fraction_bits=24  en=off  latency=0  precision=User Defined  arith_type=Unsigned  n_bits=10  bin_pt=0  quantization=Truncate  overflow=Saturate  dbl_ovrd=off  use_behavioral_HDL=off  mem_type=Distributed RAM  pipeline=off  block_type=cmult
  CMult7 : xbsIndex_r4/CMult  const=0.1  gui_display_data_type=Fixed-point  const_n_bits=20  const_bin_pt=20  float_type=Single  exp_bits=8  fraction_bits=24  en=off  latency=0  precision=User Defined  arith_type=Unsigned  n_bits=4  bin_pt=0  quantization=Truncate  overflow=Saturate  dbl_ovrd=off  use_behavioral_HDL=off  mem_type=Distributed RAM  pipeline=off  block_type=cmult
  CMult8 : xbsIndex_r4/CMult  const=10  gui_display_data_type=Fixed-point  const_n_bits=7  const_bin_pt=0  float_type=Single  exp_bits=8  fraction_bits=24  en=off  latency=0  precision=User Defined  arith_type=Unsigned  n_bits=7  bin_pt=0  quantization=Truncate  overflow=Saturate  dbl_ovrd=off  use_behavioral_HDL=off  mem_type=Distributed RAM  pipeline=off  block_type=cmult
  Vect_1 : Outport
  Vect_2 : Outport  Port=2
  Vect_3 : Outport  Port=3
  Vect_4 : Outport  Port=4
  wires:
  vector/1 -> CMult3/1, AddSub3/1
  CMult3/1 -> Vect_1/1, CMult4/1
  CMult4/1 -> AddSub3/2
  AddSub3/1 -> CMult5/1, AddSub4/1
  CMult5/1 -> Vect_2/1, CMult6/1
  CMult6/1 -> AddSub4/2
  AddSub4/1 -> AddSub5/1, CMult7/1
  CMult7/1 -> Vect_3/1, CMult8/1
  CMult8/1 -> AddSub5/2
  AddSub5/1 -> Vect_4/1

== system LF_V15_Delay_Perfect/DC_Direction_Controller/PID_Controller_ DC:LM/ID_Controller ==
  Error : Inport
  Samp_Rate : Inport  Port=2
  AddSub1 : xbsIndex_r4/AddSub  mode=Addition  use_carryin=off  use_carryout=off  en=off  latency=0  precision=Full  arith_type="Signed  (2's comp)"  n_bits=25  bin_pt=20  quantization=Truncate  overflow=Wrap  dbl_ovrd=off  use_behavioral_HDL=off  hw_selection=Fabric  pipelined=off  block_type=addsub
  Derivative : Subsystem
  Integral : Subsystem
  ID_Out : Outport
  wires:
  Samp_Rate/1 -> Integral/2(Enable), Derivative/2(Enable)
  Derivative/1(D_actuator) -> AddSub1/1
  Error/1 -> Integral/1(Err), Derivative/1(Err)
  AddSub1/1 -> ID_Out/1
  Integral/1(I Actuator) -> AddSub1/2

== system LF_V15_Delay_Perfect/DC_Direction_Controller/PID_Controller_ DC:LM/P_Controller ==
  Err : Inport
  CMult1 : xbsIndex_r4/CMult  const=Kp2  gui_display_data_type=Fixed-point  const_n_bits=2  const_bin_pt=2  float_type=Single  exp_bits=8  fraction_bits=24  en=off  latency=0  precision=User Defined  arith_type="Signed  (2's comp)"  n_bits=15  bin_pt=12  quantization=Truncate  overflow=Wrap  dbl_ovrd=off  use_behavioral_HDL=off  mem_type=Distributed RAM  pipeline=off  block_type=cmult
  Mux2 : xbsIndex_r4/Mux  inputs=2  en=off  latency=0  precision=Full  arith_type="Signed  (2's comp)"  n_bits=15  bin_pt=12  quantization=Truncate  overflow=Wrap  dbl_ovrd=off  block_type=mux
  No_Error2 : xbsIndex_r4/Constant  const=0  gui_display_data_type=Fixed-point  arith_type=Unsigned  n_bits=1  bin_pt=0  preci_type=Single  exp_width=8  frac_width=24  explicit_period=on  period=Exp_ST  equ=P=C  opselect=C  inp2=PCIN>>17  opr=+  inp1=P  carry=CIN  dbl_ovrd=off  block_type=constant
  P_Out : Outport
  tag scope: LM_PError=global
  wires:
  Err/1 -> [LM_PError], CMult1/1
  Mux2/1 -> P_Out/1
  [P_Change] -> Mux2/1
  CMult1/1 -> Mux2/3
  No_Error2/1 -> Mux2/2

== system LF_V15_Delay_Perfect/DC_Direction_Controller/PID_Controller_ DC:LM/RS_Mask_Control ==
  AddSub1 : xbsIndex_r4/AddSub  mode=Addition  use_carryin=off  use_carryout=off  en=off  latency=0  precision=Full  arith_type="Signed  (2's comp)"  n_bits=10  bin_pt=0  quantization=Truncate  overflow=Wrap  dbl_ovrd=off  use_behavioral_HDL=off  hw_selection=Fabric  pipelined=off  block_type=addsub
  AddSub3 : xbsIndex_r4/AddSub  mode=Addition  use_carryin=off  use_carryout=off  en=off  latency=0  precision=Full  arith_type="Signed  (2's comp)"  n_bits=10  bin_pt=0  quantization=Truncate  overflow=Wrap  dbl_ovrd=off  use_behavioral_HDL=off  hw_selection=Fabric  pipelined=off  block_type=addsub
  Const5 : xbsIndex_r4/Constant  const=8  gui_display_data_type=Fixed-point  arith_type=Unsigned  n_bits=4  bin_pt=0  preci_type=Single  exp_width=8  frac_width=24  explicit_period=on  period=Exp_ST  equ=P=C  opselect=C  inp2=PCIN>>17  opr=+  inp1=P  carry=CIN  dbl_ovrd=off  block_type=constant
  Delay : xbsIndex_r4/Delay  rst=off  infoeditControl=Selection of Reset will increase slice count due to use of real FFs and instead of SRLs  en=off  latency=1  dbl_ovrd=off  reg_retiming=on  block_type=delay
  Relational5 : xbsIndex_r4/Relational  mode=a<b  en=off  latency=0  dbl_ovrd=off  block_type=relational
  Scaling(-1) : xbsIndex_r4/CMult  const=-1  gui_display_data_type=Fixed-point  const_n_bits=2  const_bin_pt=0  float_type=Single  exp_bits=8  fraction_bits=24  en=off  latency=0  precision=User Defined  arith_type=Unsigned  n_bits=9  bin_pt=0  quantization=Truncate  overflow=Wrap  dbl_ovrd=off  use_behavioral_HDL=on  mem_type=Distributed RAM  pipeline=off  block_type=cmult
  RS_Mask : Outport
  tag scope: LM_T_Error=global
  wires:
  Scaling(-1)/1 -> Relational5/1, [LM_T_Error]
  Delay/1 -> RS_Mask/1
  Relational5/1 -> Delay/1
  Const5/1 -> Relational5/2
  [LM_PError] -> AddSub3/2, Scaling(-1)/1
  [LM_IError] -> AddSub1/2
  [LM_DError] -> AddSub1/1
  AddSub1/1 -> AddSub3/1

== system LF_V15_Delay_Perfect/DC_Direction_Controller/PID_Controller_ DC:RM/ID_Controller ==
  Error : Inport
  Samp_Rate : Inport  Port=2
  AddSub1 : xbsIndex_r4/AddSub  mode=Addition  use_carryin=off  use_carryout=off  en=off  latency=0  precision=Full  arith_type="Signed  (2's comp)"  n_bits=25  bin_pt=20  quantization=Truncate  overflow=Wrap  dbl_ovrd=off  use_behavioral_HDL=off  hw_selection=Fabric  pipelined=off  block_type=addsub
  Derivative : Subsystem
  Integral : Subsystem
  ID_Out : Outport
  wires:
  Integral/1(I Actuator) -> AddSub1/2
  AddSub1/1 -> ID_Out/1
  Error/1 -> Derivative/1(Err), Integral/1(Err)
  Derivative/1(D_actuator) -> AddSub1/1
  Samp_Rate/1 -> Derivative/2(Enable), Integral/2(Enable)

== system LF_V15_Delay_Perfect/DC_Direction_Controller/PID_Controller_ DC:RM/LS_Mask_Control ==
  AddSub1 : xbsIndex_r4/AddSub  mode=Addition  use_carryin=off  use_carryout=off  en=off  latency=0  precision=Full  arith_type="Signed  (2's comp)"  n_bits=10  bin_pt=0  quantization=Truncate  overflow=Wrap  dbl_ovrd=off  use_behavioral_HDL=off  hw_selection=Fabric  pipelined=off  block_type=addsub
  AddSub3 : xbsIndex_r4/AddSub  mode=Addition  use_carryin=off  use_carryout=off  en=off  latency=0  precision=Full  arith_type="Signed  (2's comp)"  n_bits=10  bin_pt=0  quantization=Truncate  overflow=Wrap  dbl_ovrd=off  use_behavioral_HDL=off  hw_selection=Fabric  pipelined=off  block_type=addsub
  Const5 : xbsIndex_r4/Constant  const=8  gui_display_data_type=Fixed-point  arith_type=Unsigned  n_bits=4  bin_pt=0  preci_type=Single  exp_width=8  frac_width=24  explicit_period=on  period=Exp_ST  equ=P=C  opselect=C  inp2=PCIN>>17  opr=+  inp1=P  carry=CIN  dbl_ovrd=off  block_type=constant
  Delay : xbsIndex_r4/Delay  rst=off  infoeditControl=Selection of Reset will increase slice count due to use of real FFs and instead of SRLs  en=off  latency=1  dbl_ovrd=off  reg_retiming=on  block_type=delay
  Relational5 : xbsIndex_r4/Relational  mode=a<b  en=off  latency=0  dbl_ovrd=off  block_type=relational
  Scaling(-1) : xbsIndex_r4/CMult  const=-1  gui_display_data_type=Fixed-point  const_n_bits=2  const_bin_pt=0  float_type=Single  exp_bits=8  fraction_bits=24  en=off  latency=0  precision=User Defined  arith_type=Unsigned  n_bits=9  bin_pt=0  quantization=Truncate  overflow=Wrap  dbl_ovrd=off  use_behavioral_HDL=on  mem_type=Distributed RAM  pipeline=off  block_type=cmult
  LS_Mask : Outport
  tag scope: RM_T_Error=global
  wires:
  AddSub1/1 -> AddSub3/1
  [RM_DError] -> AddSub1/1
  [RM_IError] -> AddSub1/2
  [RM_PError] -> AddSub3/2, Scaling(-1)/1
  Const5/1 -> Relational5/2
  Relational5/1 -> Delay/1
  Delay/1 -> LS_Mask/1
  Scaling(-1)/1 -> Relational5/1, [RM_T_Error]

== system LF_V15_Delay_Perfect/DC_Direction_Controller/PID_Controller_ DC:RM/P_Controller ==
  Err : Inport
  CMult1 : xbsIndex_r4/CMult  const=Kp2  gui_display_data_type=Fixed-point  const_n_bits=2  const_bin_pt=2  float_type=Single  exp_bits=8  fraction_bits=24  en=off  latency=0  precision=User Defined  arith_type="Signed  (2's comp)"  n_bits=15  bin_pt=12  quantization=Truncate  overflow=Wrap  dbl_ovrd=off  use_behavioral_HDL=off  mem_type=Distributed RAM  pipeline=off  block_type=cmult
  Mux2 : xbsIndex_r4/Mux  inputs=2  en=off  latency=0  precision=Full  arith_type="Signed  (2's comp)"  n_bits=15  bin_pt=12  quantization=Truncate  overflow=Wrap  dbl_ovrd=off  block_type=mux
  No_Error2 : xbsIndex_r4/Constant  const=0  gui_display_data_type=Fixed-point  arith_type=Unsigned  n_bits=1  bin_pt=0  preci_type=Single  exp_width=8  frac_width=24  explicit_period=on  period=Exp_ST  equ=P=C  opselect=C  inp2=PCIN>>17  opr=+  inp1=P  carry=CIN  dbl_ovrd=off  block_type=constant
  P_Out : Outport
  tag scope: RM_PError=global
  wires:
  Err/1 -> [RM_PError], CMult1/1
  Mux2/1 -> P_Out/1
  [P_Change] -> Mux2/1
  CMult1/1 -> Mux2/3
  No_Error2/1 -> Mux2/2
